simulink model "patt_spat"  (Simulink 6.4)
settings: Solver=FixedStepDiscrete  SolverMode=SingleTasking  StartTime=0.0  StopTime=inf  RelTol=1e-3
InitFcn:
  | vipdh_pattern;
model workspace: external: M-Code (data not in the file)
values from neighbouring files (symbols this model uses):
  pyramiding_factor = 1/str2double(get_param(model_path,'pfactor'))    [vipdh_pattern.m]
  target_dim_nopyramid = size(target_img)    [vipdh_pattern.m]
  target_img_pyramid = imresize(target_img, pyramiding_factor)    [vipdh_pattern.m]
undefined symbols (not defined in the file or in its folder): hot
libraries: vipsnks x2, viptextngfix x2, vipstatistics x2, dspwin32 x1, vipmisc x1, vipgeotforms x1, dspsnks4 x1
CloseFcn:
  | vipdh_pattern_clear;
settings Model: Creator=witek  LastModifiedBy=Administrator  ExtModeAutoUpdateStatusClock=off  ProdHWDeviceType=Specified
settings DataIOCC: LimitDataPoints=off  SaveOutput=off  SaveTime=off  SignalLoggingName=sigsOut
settings DebuggingCC: CheckExecutionContextPreStartOutputMsg=on  CheckExecutionContextRuntimeOutputMsg=on  SolverPrmCheckMsg=none  StrictBusMsg=None
settings HardwareCC: ProdHWDeviceType=Specified
settings ModelReferenceCC: UpdateModelReferenceTargets=IfOutOfDate

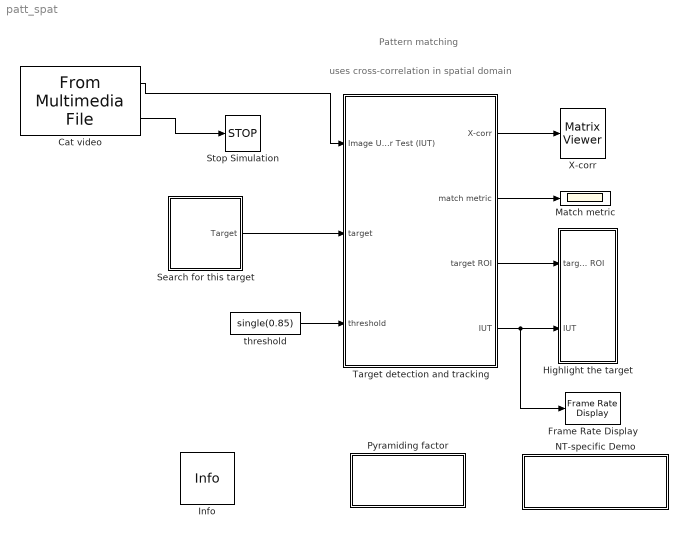
== system patt_spat ==
  note: Pattern matching
  note: uses cross-correlation in spatial domain
  Cat video : dspwin32/From Multimedia File  DialogController=dspDDGCreate  DialogControllerArgs=DataTag0  inputFilename=C:\fypthings\things2.avi  loop=on  numPlays=inf  outputStreams=Video and audio  videoDataType=uint8  audioDataType=int16  inheritSampleTime=on  userDefinedSampleTime=1/30  noAudioOutput=off  isIntensityVideo=on  outputEOF=on
  Frame Rate Display : vipsnks/Frame Rate Display  DialogController=vipDDGCreate  DialogControllerArgs=DataTag1  UpdateRate=10
  Highlight the target : Subsystem
  Info : vipmisc/Info  SystemSampleTime=-1
  Match metric : Scope
      settings: TimeRange=10  YMin=0.7  YMax=1
  NT-specific Demo : Subsystem
      settings: OpenFcn=patt
      mask Type: NT-only Demo
      mask Display: disp('Frequency-domain\nDemo')
  Pyramiding factor : Subsystem  mask(Pyramiding factor){pfactor=5}
      mask prompts: pfactor "Pyramiding factor"
      mask help:
      | The pyramiding factor is used to scale the input video so that the
      | cross-correlation is performed on a much smaller video frame thus
      | speeding up the pattern matching process.  The factor can be any
      | number from 1 to 5.  The accuracy of the match will degrade
      | proportionately to the size of the pyramiding factor.
      mask StyleString: popup(1|2|3|4|5)
      mask Display: disp('Set pyramiding\n factor')
  Search for this target : Subsystem
      mask Display: image(repmat(imread('things2_target.jpg'),[1,1,3]))
  Stop Simulation : Stop
  Target detection and tracking : Subsystem
  X-corr : dspsnks4/Matrix Viewer  DialogController=dspdialog.MatrixViewer  DialogControllerArgs=DataTag7  ImageParams=on  CMapStr=hot(256)  AxisColorbar=on  AxisParams=on  AxisOrigin=Upper left corner  XLabel=X-axis  YLabel=Y-axis  ZLabel=Z-axis  FigPos=[616 308 369 234]  AxisZoom=off
      settings: YMin=0.7  YMax=1
  threshold : Constant  Value=single(0.85)  VectorParams1D=off  OutDataType=sfix(16)  ConRadixGroup=Use specified scaling  OutScaling=2^0  SampleTime=inf  FramePeriod=inf
  wires:
  Cat video/1 -> Target detection and tracking/1(Image Under Test (IUT))
  Search for this target/1(Target) -> Target detection and tracking/2(target)
  Target detection and tracking/1(X-corr) -> X-corr/1
  Target detection and tracking/2(match metric) -> Match metric/1
  threshold/1 -> Target detection and tracking/3(threshold)
  Target detection and tracking/3(target ROI) -> Highlight the target/1(target ROI)
  Target detection and tracking/4(IUT) -> Highlight the target/2(IUT), Frame Rate Display/1
  Cat video/2 -> Stop Simulation/1

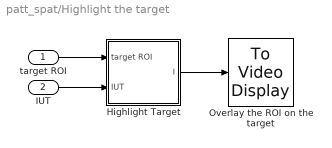
== system patt_spat/Highlight the target ==
  target ROI : Inport
  IUT : Inport  Port=2
  Highlight Target : Subsystem
  Overlay the ROI on the target : vipsnks/To Video Display  inputType=Intensity  OutputDevice=On-screen video monitor  fullScreen=off  videoWindowX=564  videoWindowY=9  saveWindowSize=off  videoWindowWidth=168  videoWindowHeight=147
  wires:
  target ROI/1 -> Highlight Target/1(target ROI)
  IUT/1 -> Highlight Target/2(IUT)
  Highlight Target/1(I) -> Overlay the ROI on the target/1

== system patt_spat/NT-specific Demo ==

== system patt_spat/Pyramiding factor ==

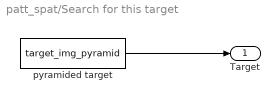
== system patt_spat/Search for this target ==
  pyramided target : Constant  Value=target_img_pyramid  VectorParams1D=off  OutDataTypeMode=single  OutDataType=sfix(16)  ConRadixGroup=Use specified scaling  OutScaling=2^0  SampleTime=inf  FramePeriod=inf
  Target : Outport
  wires:
  pyramided target/1 -> Target/1

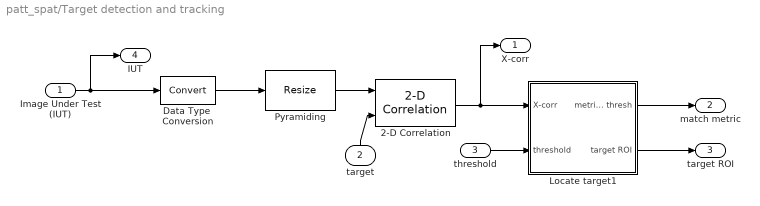
== system patt_spat/Target detection and tracking ==
  Image Under Test (IUT) : Inport
  target : Inport  Orientation=up  Port=2
  threshold : Inport  Port=3
  2-D Correlation : vipstatistics/2-D Correlation  DialogController=vipDDGCreate  DialogControllerArgs=DataTag4  outSize=Valid  normalize=on  roundingMode=Floor  overflowMode=off
  Data Type  Conversion : DataTypeConversion  OutDataTypeMode=single  SaturateOnIntegerOverflow=on  RndMeth=Zero
  Locate target1 : Subsystem
  Pyramiding : vipgeotforms/Resize  DialogController=vipDDGCreate  DialogControllerArgs=DataTag6  specify=Output size as a percentage of input size  rfactor=pyramiding_factor*100  outCols=25  outRows=25  outRowsCols=[25 35]  interp_method=Bicubic  antialias=off  roundingMode=Floor  overflowMode=off
  X-corr : Outport
  match metric : Outport  Port=2
  target ROI : Outport  Port=3
  IUT : Outport  Port=4
  wires:
  Pyramiding/1 -> 2-D Correlation/1
  threshold/1 -> Locate target1/2(threshold)
  Data Type  Conversion/1 -> Pyramiding/1
  Locate target1/1(metric and thresh) -> match metric/1
  Locate target1/2(target ROI) -> target ROI/1
  Image Under Test (IUT)/1 -> Data Type  Conversion/1, IUT/1
  target/1 -> 2-D Correlation/2
  2-D Correlation/1 -> X-corr/1, Locate target1/1(X-corr)

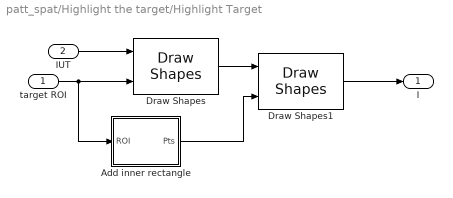
== system patt_spat/Highlight the target/Highlight Target ==
  target ROI : Inport
  IUT : Inport  Port=2
  Add inner rectangle : Subsystem
  Draw Shapes : viptextngfix/Draw Shapes  DialogController=vipDDGCreate  DialogControllerArgs=DataTag2  inType=Intensity  shape=Rectangles  fill=off  display=Black  intensity=200  color=[200 255 100]  opacity=0.6  viewport=Entire image  antialiasing=off
  Draw Shapes1 : viptextngfix/Draw Shapes  DialogController=vipDDGCreate  DialogControllerArgs=DataTag3  inType=Intensity  shape=Rectangles  fill=off  display=White  intensity=200  color=[200 255 100]  opacity=0.6  viewport=Entire image  antialiasing=off
  I : Outport
  wires:
  IUT/1 -> Draw Shapes/1
  target ROI/1 -> Draw Shapes/2, Add inner rectangle/1(ROI)
  Draw Shapes/1 -> Draw Shapes1/1
  Add inner rectangle/1(Pts) -> Draw Shapes1/2
  Draw Shapes1/1 -> I/1

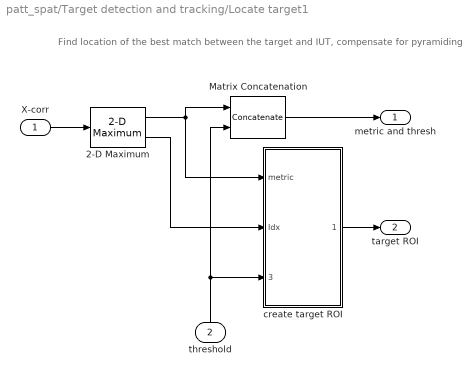
== system patt_spat/Target detection and tracking/Locate target1 ==
  note: Find location of the best match
      | between the target and IUT,
      | compensate for pyramiding
  X-corr : Inport
  threshold : Inport  Orientation=up  Port=2
  2-D Maximum : vipstatistics/2-D Maximum  DialogController=dspDDGCreate  DialogControllerArgs=DataTag5  fcn=Value and Index  reset=None  roundingMode=Nearest  overflowMode=off
  Matrix Concatenation : Concatenate  Mode=Horizontal matrix concatenation
  create target ROI : Subsystem
  metric and thresh : Outport
  target ROI : Outport  Port=2
  wires:
  threshold/1 -> create target ROI/3(threshold), Matrix Concatenation/2
  2-D Maximum/1 -> create target ROI/1(metric), Matrix Concatenation/1
  X-corr/1 -> 2-D Maximum/1
  create target ROI/1(target ROI) -> target ROI/1
  2-D Maximum/2 -> create target ROI/2(Idx)
  Matrix Concatenation/1 -> metric and thresh/1

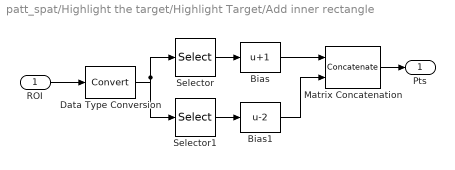
== system patt_spat/Highlight the target/Highlight Target/Add inner rectangle ==
  ROI : Inport
  Bias : Bias  Bias=1
  Bias1 : Bias  Bias=-2
  Data Type Conversion : DataTypeConversion  OutDataTypeMode=int32
  Matrix Concatenation : Concatenate  Mode=Horizontal matrix concatenation
  Selector : Selector  IndexMode=Zero-based  Elements=[0 1]  InputPortWidth=4
  Selector1 : Selector  IndexMode=Zero-based  Elements=[2 3]  InputPortWidth=4
  Pts : Outport
  wires:
  Selector/1 -> Bias/1
  Selector1/1 -> Bias1/1
  Bias/1 -> Matrix Concatenation/1
  Bias1/1 -> Matrix Concatenation/2
  Data Type Conversion/1 -> Selector/1, Selector1/1
  ROI/1 -> Data Type Conversion/1
  Matrix Concatenation/1 -> Pts/1

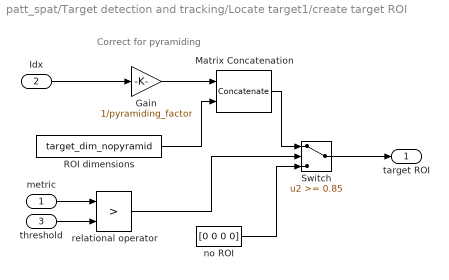
== system patt_spat/Target detection and tracking/Locate target1/create target ROI ==
  note: Correct for
      |  pyramiding
  metric : Inport
  Idx : Inport  Port=2
  threshold : Inport  Port=3
  Gain : Gain  Gain=1/pyramiding_factor  ParameterDataTypeMode=Specify via dialog  ParameterDataType=float('single')  ParameterScalingMode=Best Precision: Element-wise  ParameterScaling=2^-16  RndMeth=Nearest  SaturateOnIntegerOverflow=on
  Matrix Concatenation : Concatenate  Mode=Horizontal matrix concatenation
  ROI dimensions : Constant  Value=target_dim_nopyramid  VectorParams1D=off  OutDataTypeMode=uint32  OutDataType=sfix(16)  ConRadixGroup=Use specified scaling  OutScaling=2^0  SampleTime=inf  FramePeriod=inf
  Switch : Switch  Threshold=0.85
  no ROI : Constant  Value=[0 0 0 0]  OutDataTypeMode=uint32  OutDataType=sfix(16)  ConRadixGroup=Use specified scaling  OutScaling=2^0  SampleTime=inf  FramePeriod=inf
  relational operator : RelationalOperator  Operator=>  LogicOutDataTypeMode=Boolean  ZeroCross=off
  target ROI : Outport
  wires:
  ROI dimensions/1 -> Matrix Concatenation/2
  Switch/1 -> target ROI/1
  no ROI/1 -> Switch/3
  metric/1 -> relational operator/1
  threshold/1 -> relational operator/2
  relational operator/1 -> Switch/2
  Gain/1 -> Matrix Concatenation/1
  Idx/1 -> Gain/1
  Matrix Concatenation/1 -> Switch/1
